simulink model "NETWORK"  (Simulink 7.3)
settings: Solver=ode45  StartTime=0.0  StopTime=.6  RelTol=1e-3
undefined symbols (not defined in the file or in its folder): x
libraries: powerlib x218, powerlib_extras x125
(part 3 of 3)

== matlab function Subsystem3/1 constant power/Embedded MATLAB Function1 ==
  data: b input double; y output double
function y = fcn(b)
%#eml

y = [1/sqrt(3) 1/sqrt(3) 1/sqrt(3); sqrt(2)/sqrt(3) -sqrt(2)/(2*sqrt(3)) -sqrt(2)/(2*sqrt(3)); 0 1/sqrt(2) -1/sqrt(2)]*b;

== matlab function Subsystem3/1 constant power/Embedded MATLAB Function3 ==
  data: h input double; y output double
function y = fcn(h)
%#eml

y =[1/sqrt(3) sqrt(2)/sqrt(3) 0 ;1/sqrt(3) -sqrt(2)/(2*sqrt(3)) 1/sqrt(2) ;1/sqrt(3) -sqrt(2)/(2*sqrt(3)) -1/sqrt(2)]*h;

== matlab function Subsystem3/1 constant power/Embedded MATLAB Function4 ==
  data: a input double; y output double
function y = fcn(a)
% #eml
if (a(2)^2+a(3)^2)==0
    y=[0; 0;0];
else
y =-[0;a(2);a(3)]*(a(4)/(a(2)^2+a(3)^2))+[a(5);a(6);a(7)];
end

== matlab function Subsystem3/2 unity PF/Embedded MATLAB Function ==
  data: a input double; y output double
function y = fcn(a)
%#eml

y =[1/sqrt(3) 1/sqrt(3) 1/sqrt(3); sqrt(2)/sqrt(3) -sqrt(2)/(2*sqrt(3)) -sqrt(2)/(2*sqrt(3)); 0 1/sqrt(2) -1/sqrt(2)]*a;

== matlab function Subsystem4/1 constant power/Embedded MATLAB Function3 ==
  data: h input double; y output double
function y = fcn(h)
%#eml

y =[1/sqrt(3) sqrt(2)/sqrt(3) 0 ;1/sqrt(3) -sqrt(2)/(2*sqrt(3)) 1/sqrt(2) ;1/sqrt(3) -sqrt(2)/(2*sqrt(3)) -1/sqrt(2)]*h;

== matlab function Subsystem4/1 constant power/Embedded MATLAB Function4 ==
  data: a input double; y output double
function y = fcn(a)
% #eml
if (a(2)^2+a(3)^2)==0
    y=[0; 0;0];
else
y =-[0;a(2);a(3)]*(a(4)/(a(2)^2+a(3)^2))+[a(5);a(6);a(7)];
end

== matlab function Subsystem4/2 unity PF/Embedded MATLAB Function ==
  data: a input double; y output double
function y = fcn(a)
%#eml

y =[1/sqrt(3) 1/sqrt(3) 1/sqrt(3); sqrt(2)/sqrt(3) -sqrt(2)/(2*sqrt(3)) -sqrt(2)/(2*sqrt(3)); 0 1/sqrt(2) -1/sqrt(2)]*a;

== matlab function Subsystem4/2 unity PF/Embedded MATLAB Function1 ==
  data: b input double; y output double
function y = fcn(b)
%#eml

y = [1/sqrt(3) 1/sqrt(3) 1/sqrt(3); sqrt(2)/sqrt(3) -sqrt(2)/(2*sqrt(3)) -sqrt(2)/(2*sqrt(3)); 0 1/sqrt(2) -1/sqrt(2)]*b;

== matlab function Subsystem4/2 unity PF/Embedded MATLAB Function2 ==
  data: a input double; y output double
function y = fcn(a)
% #eml

y =(a(1)^2+a(2)^2+a(3)^2);

== matlab function Subsystem4/2 unity PF/Embedded MATLAB Function3 ==
  data: h input double; y output double
function y = fcn(h)
%#eml

y =[1/sqrt(3) sqrt(2)/sqrt(3) 0 ;1/sqrt(3) -sqrt(2)/(2*sqrt(3)) 1/sqrt(2) ;1/sqrt(3) -sqrt(2)/(2*sqrt(3)) -1/sqrt(2)]*h;

== matlab function Subsystem4/2 unity PF/Embedded MATLAB Function4 ==
  data: a input double; y output double
function y = fcn(a)
% #eml
if a(7)<10
    y=[0; 0;0];
else
y =[a(1);a(2);a(3)]-[a(4);a(5);a(6)]*((a(8)/a(7)));
end

== matlab function Subsystem4/3 balanced currents /Embedded MATLAB Function ==
  data: u input double; iL_0dq output double
function iL_0dq = fcn(u)
%#eml

iL_0dq =[1/sqrt(3) 1/sqrt(3) 1/sqrt(3); sqrt(2)/sqrt(3) -sqrt(2)/(2*sqrt(3)) -sqrt(2)/(2*sqrt(3)); 0 1/sqrt(2) -1/sqrt(2)]*u;

== matlab function Subsystem4/3 balanced currents /Embedded MATLAB Function2 ==
  data: u input double; iL_0dq output double
function iL_0dq = fcn(u)
%#eml
if u(7)==0
    iL_0dq=[0;0;0];
else
iL_0dq =[u(1);u(2);u(3)]-(u(8)/u(7))*[0;u(5);u(6)];
end

== matlab function Subsystem3/2 unity PF/Embedded MATLAB Function1 ==
  data: b input double; y output double
function y = fcn(b)
%#eml

y = [1/sqrt(3) 1/sqrt(3) 1/sqrt(3); sqrt(2)/sqrt(3) -sqrt(2)/(2*sqrt(3)) -sqrt(2)/(2*sqrt(3)); 0 1/sqrt(2) -1/sqrt(2)]*b;

== matlab function Subsystem3/2 unity PF/Embedded MATLAB Function2 ==
  data: a input double; y output double
function y = fcn(a)
% #eml

y =(a(1)^2+a(2)^2+a(3)^2);

== matlab function Subsystem3/2 unity PF/Embedded MATLAB Function3 ==
  data: h input double; y output double
function y = fcn(h)
%#eml

y =[1/sqrt(3) sqrt(2)/sqrt(3) 0 ;1/sqrt(3) -sqrt(2)/(2*sqrt(3)) 1/sqrt(2) ;1/sqrt(3) -sqrt(2)/(2*sqrt(3)) -1/sqrt(2)]*h;

== matlab function Subsystem3/2 unity PF/Embedded MATLAB Function4 ==
  data: a input double; y output double
function y = fcn(a)
% #eml
if a(7)<10
    y=[0; 0;0];
else
y =[a(1);a(2);a(3)]-[a(4);a(5);a(6)]*((a(8)/a(7)));
end

== matlab function Subsystem3/3 balanced currents /Embedded MATLAB Function ==
  data: u input double; iL_0dq output double
function iL_0dq = fcn(u)
%#eml

iL_0dq =[1/sqrt(3) 1/sqrt(3) 1/sqrt(3); sqrt(2)/sqrt(3) -sqrt(2)/(2*sqrt(3)) -sqrt(2)/(2*sqrt(3)); 0 1/sqrt(2) -1/sqrt(2)]*u;

== matlab function Subsystem3/3 balanced currents /Embedded MATLAB Function2 ==
  data: u input double; iL_0dq output double
function iL_0dq = fcn(u)
%#eml
if u(7)==0
    iL_0dq=[0;0;0];
else
iL_0dq =[u(1);u(2);u(3)]-(u(8)/u(7))*[0;u(5);u(6)];
end

== matlab function Subsystem3/3 balanced currents /Embedded MATLAB Function3 ==
  data: u input double; y output double
function y = fcn(u)
%#eml

y =[1/sqrt(3) sqrt(2)/sqrt(3) 0 ;1/sqrt(3) -sqrt(2)/(2*sqrt(3)) 1/sqrt(2) ;1/sqrt(3) -sqrt(2)/(2*sqrt(3)) -1/sqrt(2)]*u;

== matlab function PF17 ==
  data: u input double; y output double
function y = fcn(u)
%#eml

y = cos(atan(u(2)/u(1)));

== matlab function PF18 ==
  data: u input double; y output double
function y = fcn(u)
%#eml

y = cos(atan(u(2)/u(1)));

== matlab function Subsystem5/1 constant power/Embedded MATLAB Function ==
  data: a input double; y output double
function y = fcn(a)
%#eml

y =[1/sqrt(3) 1/sqrt(3) 1/sqrt(3); sqrt(2)/sqrt(3) -sqrt(2)/(2*sqrt(3)) -sqrt(2)/(2*sqrt(3)); 0 1/sqrt(2) -1/sqrt(2)]*a;

== matlab function Subsystem5/1 constant power/Embedded MATLAB Function1 ==
  data: b input double; y output double
function y = fcn(b)
%#eml

y = [1/sqrt(3) 1/sqrt(3) 1/sqrt(3); sqrt(2)/sqrt(3) -sqrt(2)/(2*sqrt(3)) -sqrt(2)/(2*sqrt(3)); 0 1/sqrt(2) -1/sqrt(2)]*b;

== matlab function Subsystem5/1 constant power/Embedded MATLAB Function3 ==
  data: h input double; y output double
function y = fcn(h)
%#eml

y =[1/sqrt(3) sqrt(2)/sqrt(3) 0 ;1/sqrt(3) -sqrt(2)/(2*sqrt(3)) 1/sqrt(2) ;1/sqrt(3) -sqrt(2)/(2*sqrt(3)) -1/sqrt(2)]*h;

== matlab function Subsystem5/1 constant power/Embedded MATLAB Function4 ==
  data: a input double; y output double
function y = fcn(a)
% #eml
if (a(2)^2+a(3)^2)==0
    y=[0; 0;0];
else
y =-[0;a(2);a(3)]*(a(4)/(a(2)^2+a(3)^2))+[a(5);a(6);a(7)];
end

== matlab function Subsystem5/2 unity PF/Embedded MATLAB Function ==
  data: a input double; y output double
function y = fcn(a)
%#eml

y =[1/sqrt(3) 1/sqrt(3) 1/sqrt(3); sqrt(2)/sqrt(3) -sqrt(2)/(2*sqrt(3)) -sqrt(2)/(2*sqrt(3)); 0 1/sqrt(2) -1/sqrt(2)]*a;

== matlab function Subsystem5/2 unity PF/Embedded MATLAB Function1 ==
  data: b input double; y output double
function y = fcn(b)
%#eml

y = [1/sqrt(3) 1/sqrt(3) 1/sqrt(3); sqrt(2)/sqrt(3) -sqrt(2)/(2*sqrt(3)) -sqrt(2)/(2*sqrt(3)); 0 1/sqrt(2) -1/sqrt(2)]*b;

== matlab function Subsystem5/2 unity PF/Embedded MATLAB Function2 ==
  data: a input double; y output double
function y = fcn(a)
% #eml

y =(a(1)^2+a(2)^2+a(3)^2);

== matlab function Subsystem5/2 unity PF/Embedded MATLAB Function3 ==
  data: h input double; y output double
function y = fcn(h)
%#eml

y =[1/sqrt(3) sqrt(2)/sqrt(3) 0 ;1/sqrt(3) -sqrt(2)/(2*sqrt(3)) 1/sqrt(2) ;1/sqrt(3) -sqrt(2)/(2*sqrt(3)) -1/sqrt(2)]*h;

== matlab function Subsystem5/2 unity PF/Embedded MATLAB Function4 ==
  data: a input double; y output double
function y = fcn(a)
% #eml
if a(7)<10
    y=[0; 0;0];
else
y =[a(1);a(2);a(3)]-[a(4);a(5);a(6)]*((a(8)/a(7)));
end

== matlab function Subsystem5/3 balanced currents /Embedded MATLAB Function ==
  data: u input double; iL_0dq output double
function iL_0dq = fcn(u)
%#eml

iL_0dq =[1/sqrt(3) 1/sqrt(3) 1/sqrt(3); sqrt(2)/sqrt(3) -sqrt(2)/(2*sqrt(3)) -sqrt(2)/(2*sqrt(3)); 0 1/sqrt(2) -1/sqrt(2)]*u;

== matlab function Subsystem4/3 balanced currents /Embedded MATLAB Function3 ==
  data: u input double; y output double
function y = fcn(u)
%#eml

y =[1/sqrt(3) sqrt(2)/sqrt(3) 0 ;1/sqrt(3) -sqrt(2)/(2*sqrt(3)) 1/sqrt(2) ;1/sqrt(3) -sqrt(2)/(2*sqrt(3)) -1/sqrt(2)]*u;

== matlab function Subsystem5/3 balanced currents /Embedded MATLAB Function2 ==
  data: u input double; iL_0dq output double
function iL_0dq = fcn(u)
%#eml
if u(7)==0
    iL_0dq=[0;0;0];
else
iL_0dq =[u(1);u(2);u(3)]-(u(8)/u(7))*[0;u(5);u(6)];
end

== matlab function Subsystem5/3 balanced currents /Embedded MATLAB Function3 ==
  data: u input double; y output double
function y = fcn(u)
%#eml

y =[1/sqrt(3) sqrt(2)/sqrt(3) 0 ;1/sqrt(3) -sqrt(2)/(2*sqrt(3)) 1/sqrt(2) ;1/sqrt(3) -sqrt(2)/(2*sqrt(3)) -1/sqrt(2)]*u;
